simulink model "Ejer1_EcVanDerPol"  (R2023b)
settings: Solver=VariableStepAuto  StartTime=0  StopTime=20  RelTol=1e-3
values from neighbouring files (symbols this model uses):
  dx0 = 0.25    [plantilla_sistemas_continuos.m]
  x0 = 1    [plantilla_sistemas_continuos.m]
settings Model: Creator=alfre  LastModifiedBy=alfre

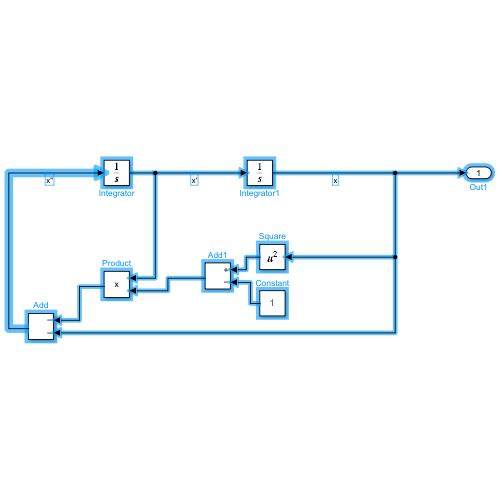
[thumbnail: Simulink's stored preview of the top-level diagram]
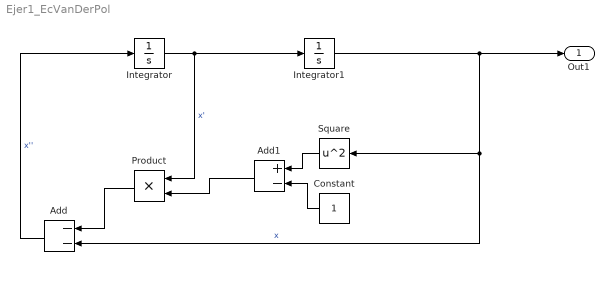
== system Ejer1_EcVanDerPol ==
  Add : Sum  Inputs=--
  Add1 : Sum  Inputs=+-
  Constant : Constant
  Integrator : Integrator  InitialCondition=dx0
  Integrator1 : Integrator  InitialCondition=x0
  Product : Product
  Square : Math  Operator=square
  Out1 : Outport
  wires:
  Integrator/1 -> Product/1, Integrator1/1  "x'"
  Add/1 -> Integrator/1  "x''"
  Integrator1/1 -> Out1/1, Square/1, Add/2  "x"
  Square/1 -> Add1/1
  Constant/1 -> Add1/2
  Product/1 -> Add/1
  Add1/1 -> Product/2
